simulink subsystem "snake_counter"  (R2022a)
settings: Solver=VariableStepAuto  StartTime=0.0  StopTime=1e-6  RelTol=1e-3
settings Model: DefaultTestHarness=snake_counter_harness  Creator=andre  LastModifiedBy=andre

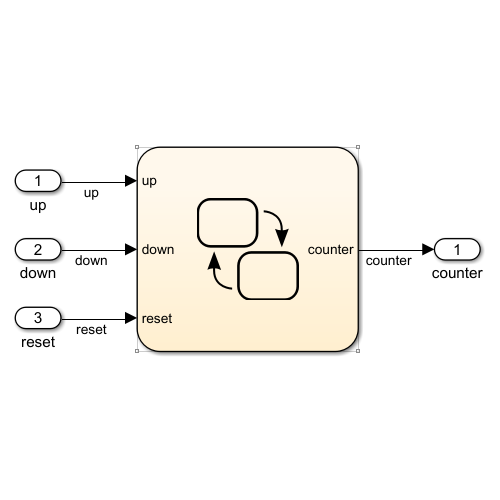
[thumbnail: Simulink's stored preview of the top-level diagram]
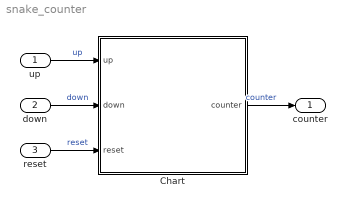
== system snake_counter ==
  up : Inport  OutDataTypeStr=boolean  PortDimensions=1
  down : Inport  Port=2  OutDataTypeStr=boolean  PortDimensions=1
  reset : Inport  Port=3  OutDataTypeStr=boolean  PortDimensions=1
  Chart : Stateflow chart  TreatAsAtomicUnit=on
  counter : Outport  OutDataTypeStr=fixdt(1,5,0)  PortDimensions=1
  wires:
  up/1 -> Chart/1(up)  "up"
  down/1 -> Chart/2(down)  "down"
  reset/1 -> Chart/3(reset)  "reset"
  Chart/1(counter) -> counter/1  "counter"

== stateflow chart snake_counter/Chart ==
  state IDLE
    en, du:
    counter = fi(1,1,5,0);
  state UP
    en:
    if counter == 9
    counter = fi(1,1,5,0);
    end
  state DOWN
    en:
    if counter == 0
    counter = fi(8,1,5,0);
    end
  (default) -> IDLE
  UP -> UP [order 2] : [up]{counter = fi(counter + fi(1,0,1,0),1,5,0);}
  UP -> IDLE [order 1] : [reset]
  IDLE -> UP : [up]{counter = fi(counter + fi(1,0,1,0),1,5,0);}
  UP -> DOWN [order 3] : [down]{counter = fi(counter - fi(1,0,1,0),1,5,0);}
  DOWN -> UP [order 3] : [up]{counter = fi(counter + fi(1,0,1,0),1,5,0);}
  DOWN -> DOWN [order 2] : [down]{counter = fi(counter - fi(1,0,1,0),1,5,0);}
  DOWN -> IDLE [order 1] : [reset]
  data: up input; down input; reset input; counter output
